simulink model "controller"  (R2025a)
settings: Solver=VariableStepAuto  StartTime=0.0  StopTime=20  RelTol=1e-3
values from neighbouring files (symbols this model uses):
  qd = [0 5.20948749525e-05 0.00020837949981 0.000468853874573 0.000833517999241 0.00130237187381 0.00187541549829 0.00255264887267 0.00333407199696 0.00421968487116 0.00520948749525 0.00630347986926 ... (2700 elements, 450x6)]    [dq.mat]
undefined symbols (not defined in the file or in its folder): D, ddqd, dqd, new_time, Q, rou
(part 1 of 2)
settings Model: Creator=CYX  LastModifiedBy=yxlewis
settings DebuggingCC: ParameterPrecisionLossMsg=none  UnderSpecifiedDimensionMsg=warning
settings RTWCC: GPUComputeCapability=3.5
settings SimscapeCC: SimscapeLogDecimation=1  SimscapeLogDataHistory=5000

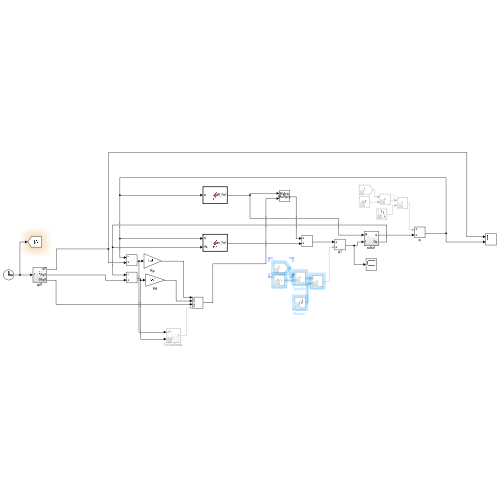
[thumbnail: Simulink's stored preview of the top-level diagram]
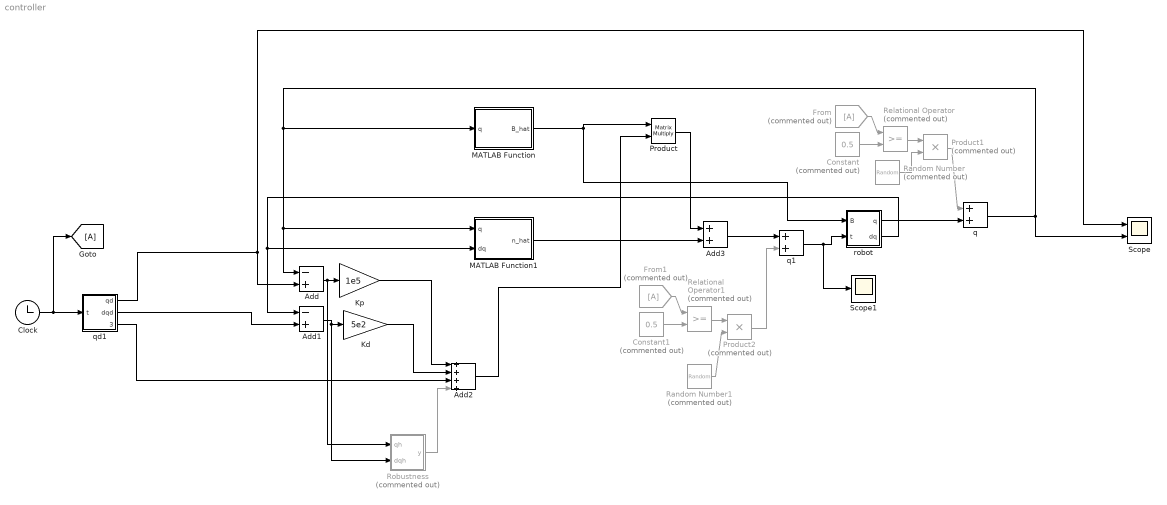
== system controller ==
  Add : Sum  Inputs=-+
  Add1 : Sum  Inputs=-+
  Add2 : Sum  Inputs=++++
  Add3 : Sum
  Clock : Clock
  Constant : Constant  Commented=on  Value=0.5
  Constant1 : Constant  Commented=on  Value=0.5
  From : From  Commented=on
  From1 : From  Commented=on
  Goto : Goto
  Kd : Gain  Gain=5e2
  Kp : Gain  Gain=1e5
  MATLAB Function : MATLAB Function  TreatAsAtomicUnit=on
  MATLAB Function1 : MATLAB Function  TreatAsAtomicUnit=on
  Product : Product  Multiplication=Matrix(*)
  Product1 : Product  Commented=on
  Product2 : Product  Commented=on
  Random Number : RandomNumber  Commented=on  Variance=1e-4  SampleTime=1e-2
  Random Number1 : RandomNumber  Commented=on  Variance=1e-4  SampleTime=1e-2
  Relational Operator : RelationalOperator  Commented=on  OutDataTypeStr=boolean  RndMeth=Simplest  InputSameDT=off
  Relational Operator1 : RelationalOperator  Commented=on  OutDataTypeStr=boolean  RndMeth=Simplest  InputSameDT=off
  Robustness : Subsystem  Commented=on
  Scope : Scope  NumInputPorts=2
      settings: ActiveDisplayYMinimum=-4.68170124056776  ActiveDisplayYMaximum=3.2186322366566769
  Scope1 : Scope
      settings: ActiveDisplayYMinimum=-244.17864380949288  ActiveDisplayYMaximum=369.16272311248588
  q : Sum
  q1 : Sum
  qd1 : Subsystem
  robot : Subsystem
  wires:
  qd1/3(ddqd) -> Add2/3
  Robustness/1(y) -> Add2/4
  Add2/1 -> Product/2
  Kp/1 -> Add2/1
  Add/1 -> Robustness/1(qh), Kp/1
  Product/1 -> Add3/1
  qd1/2(dqd) -> Add1/2
  MATLAB Function/1(B_hat) -> Product/1, robot/1(B)
  qd1/1(qd) -> Scope/1, Add/2
  Add1/1 -> Robustness/2(dqh), Kd/1
  Kd/1 -> Add2/2
  MATLAB Function1/1(n_hat) -> Add3/2
  Clock/1 -> qd1/1(t), Goto/1
  robot/2(dq) -> Add1/1, MATLAB Function1/2(dq)
  robot/1(q) -> q/2
  q/1 -> Scope/2, MATLAB Function/1(q), MATLAB Function1/1(q), Add/1
  Add3/1 -> q1/1
  q1/1 -> Scope1/1, robot/2(t)
  Constant/1 -> Relational Operator/2
  From/1 -> Relational Operator/1
  Relational Operator/1 -> Product1/1
  Random Number/1 -> Product1/2
  Product1/1 -> q/1
  Relational Operator1/1 -> Product2/1
  From1/1 -> Relational Operator1/1
  Constant1/1 -> Relational Operator1/2
  Random Number1/1 -> Product2/2
  Product2/1 -> q1/2

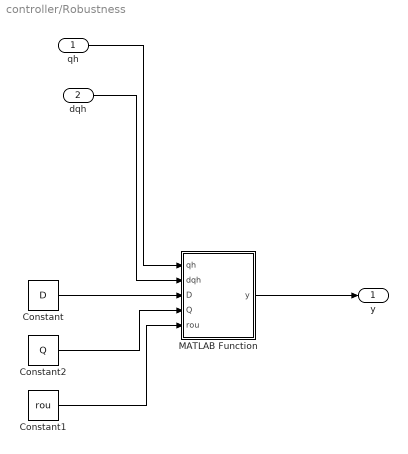
== system controller/Robustness ==
  qh : Inport
  dqh : Inport  Port=2
  Constant : Constant  Value=D
  Constant1 : Constant  Value=rou
  Constant2 : Constant  Value=Q
  MATLAB Function : MATLAB Function  TreatAsAtomicUnit=on
  y : Outport
  wires:
  Constant2/1 -> MATLAB Function/4(Q)
  dqh/1 -> MATLAB Function/2(dqh)
  qh/1 -> MATLAB Function/1(qh)
  MATLAB Function/1(y) -> y/1
  Constant/1 -> MATLAB Function/3(D)
  Constant1/1 -> MATLAB Function/5(rou)

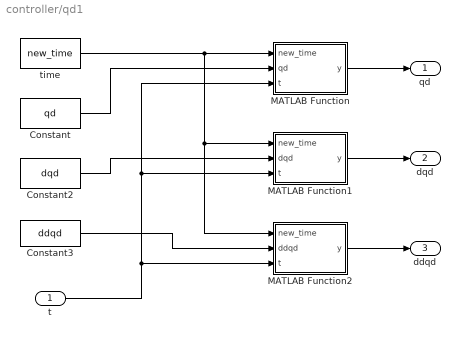
== system controller/qd1 ==
  t : Inport
  Constant : Constant  Value=qd
  Constant2 : Constant  Value=dqd
  Constant3 : Constant  Value=ddqd
  MATLAB Function : MATLAB Function  TreatAsAtomicUnit=on
  MATLAB Function1 : MATLAB Function  TreatAsAtomicUnit=on
  MATLAB Function2 : MATLAB Function  TreatAsAtomicUnit=on
  time : Constant  Value=new_time
  qd : Outport  PortDimensions=6*1
  dqd : Outport  Port=2  PortDimensions=6*1
  ddqd : Outport  Port=3  PortDimensions=6*1
  wires:
  time/1 -> MATLAB Function2/1(new_time), MATLAB Function1/1(new_time), MATLAB Function/1(new_time)
  Constant/1 -> MATLAB Function/2(qd)
  t/1 -> MATLAB Function2/3(t), MATLAB Function1/3(t), MATLAB Function/3(t)
  Constant2/1 -> MATLAB Function1/2(dqd)
  Constant3/1 -> MATLAB Function2/2(ddqd)
  MATLAB Function/1(y) -> qd/1
  MATLAB Function1/1(y) -> dqd/1
  MATLAB Function2/1(y) -> ddqd/1

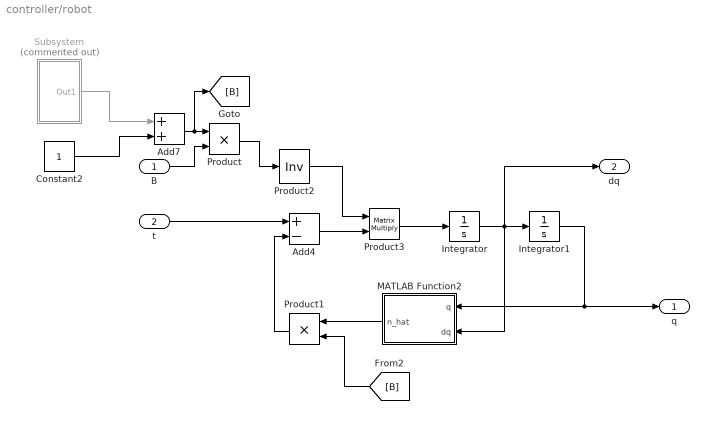
== system controller/robot ==
  B : Inport
  t : Inport  Port=2
  Add4 : Sum  Inputs=+-
  Add7 : Sum
  Constant2 : Constant
  Integrator : Integrator
  Integrator1 : Integrator
  MATLAB Function2 : MATLAB Function  TreatAsAtomicUnit=on
  Product : Product
  Product1 : Product
  Product2 : Product  Inputs=/  Multiplication=Matrix(*)
  Product3 : Product  Multiplication=Matrix(*)
  Subsystem : Subsystem  Commented=on
  q : Outport
  dq : Outport  Port=2
  wires:
  Integrator/1 -> dq/1, MATLAB Function2/2(dq), Integrator1/1
  t/1 -> Add4/1
  Product3/1 -> Integrator/1
  Integrator1/1 -> q/1, MATLAB Function2/1(q)
  Product2/1 -> Product3/1
  Add4/1 -> Product3/2
  MATLAB Function2/1(n_hat) -> Product1/1
  Product1/1 -> Add4/2
  Product/1 -> Product2/1
  Constant2/1 -> Add7/2
  Add7/1 -> [B], Product/1
  B/1 -> Product/2
  [B] -> Product1/2
  Subsystem/1(Out1) -> Add7/1

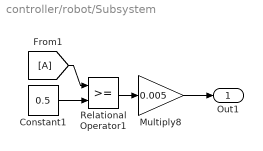
== system controller/robot/Subsystem ==
  Constant1 : Constant  Value=0.5
  From1 : From
  Multiply8 : Gain  Gain=0.005
  Relational Operator1 : RelationalOperator  OutDataTypeStr=boolean  RndMeth=Simplest  InputSameDT=off
  Out1 : Outport
  wires:
  From1/1 -> Relational Operator1/1
  Constant1/1 -> Relational Operator1/2
  Relational Operator1/1 -> Multiply8/1
  Multiply8/1 -> Out1/1

== matlab function controller/MATLAB Function1 ==
  data: q input size=6*1; n_hat output size=6*1; dq input size=6*1
function n_hat = fcn(q, dq)
th = q;
dth = dq;
th1 = th(1); th2 = th(2); th3 = th(3); th4 = th(4); th5 = th(5); th6 = th(6);
dth1 = dth(1); dth2 = dth(2); dth3 = dth(3); dth4 = dth(4); dth5 = dth(5); dth6 = dth(6);
% % ddth1 = ddth(1); ddth2 = ddth(2); ddth3 = ddth(3); ddth4 = ddth(4); ddth5 = ddth(5); ddth6 = ddth(6);

G = [0;
    (1866843*sin(th2 - th3 + th4 + th5))/2000000 - (795688119*sin(th2 - th3))/25000000 - (1866843*sin(th2 - th3 + th4 - th5))/2000000 - (40439763*sin(th2 - th3 + th4))/6250000 - (689642019*sin(th2))/12500000;
     (795688119*sin(th2 - th3))/25000000 - (1866843*sin(th2 - th3 + th4 + th5))/2000000 + (1866843*sin(th2 - th3 + th4 - th5))/2000000 + (40439763*sin(th2 - th3 + th4))/6250000;
     (1866843*sin(th2 - th3 + th4 + th5))/2000000 - (1866843*sin(th2 - th3 + th4 - th5))/2000000 - (40439763*sin(th2 - th3 + th4))/6250000;
     (1866843*sin(th2 - th3 + th4 + th5))/2000000 + (1866843*sin(th2 - th3 + th4 - th5))/2000000;
     0];

C = [(138917031*dth2^2*sin(th2))/250000000 - (5709*dth2^2*sin(th2 - th3 + th4 + th5))/2500000 - (5709*dth3^2*sin(th2 - th3 + th4 + th5))/2500000 - (5709*dth4^2*sin(th2 - th3 + th4 + th5))/2500000 - (173173*dth5^2*sin(th2 - th3 + th4 + th5))/5000000 + (2438609*dth2^2*sin(th2 - th3))/6250000 + (2438609*dth3^2*sin(th2 - th3))/6250000 + (378697*dth2^2*sin(th2 - th5))/10000000 - (378697*dth5^2*sin(th2 - th5))/10000000 + (173173*dth2^2*sin(th2 - th3 + th4 - th5))/5000000 + (2389*dth2^2*sin(th2 - th3 + th4 - 2*th5))/1250000 - (2389*dth2^2*sin(th2 - th3 + th4 + 2*th5))/1250000 + (173173*dth3^2*sin(th2 - th3 + th4 - th5))/5000000 + (2389*dth3^2*sin(th2 - th3 + th4 - 2*th5))/1250000 - (2389*dth3^2*sin(th2 - th3 + th4 + 2*th5))/1250000 + (173173*dth4^2*sin(th2 - th3 + th4 - th5))/5000000 + (2389*dth4^2*sin(th2 - th3 + th4 - 2*th5))/1250000 - (2389*dth4^2*sin(th2 - th3 + th4 + 2*th5))/1250000 + (5709*dth5^2*sin(th2 - th3 + th4 - th5))/2500000 + (3998631*dth2^2*sin(th2 - th3 + th4))/31250000 + (17127*dth2^2*sin(th2 - th3 + th5))/500000 - (17127*dth2^2*sin(th3 - th2 + th5))/500000 + (3998631*dth3^2*sin(th2 - th3 + th4))/31250000 + (17127*dth3^2*sin(th2 - th3 + th5))/500000 - (17127*dth3^2*sin(th3 - th2 + th5))/500000 + (3998631*dth4^2*sin(th2 - th3 + th4))/31250000 - (17127*dth5^2*sin(th2 - th3 + th5))/500000 + (17127*dth5^2*sin(th3 - th2 + th5))/500000 + (378697*dth2^2*sin(th2 + th5))/10000000 - (378697*dth5^2*sin(th2 + th5))/10000000 - (161408701*dth1*dth3*sin(th3))/125000000 - (371007*dth1*dth4*sin(th4))/1562500 - (184591*dth1*dth5*sin(th5))/2500000 + (8203377*dth1*dth2*sin(2*th2 - th3 + th4))/15625000 + (371007*dth1*dth2*sin(2*th2 - 2*th3 + th4))/781250 - (8203377*dth1*dth3*sin(2*th2 - th3 + th4))/31250000 - (371007*dth1*dth3*sin(2*th2 - 2*th3 + th4))/781250 + (8203377*dth1*dth4*sin(2*th2 - th3 + th4))/31250000 + (371007*dth1*dth4*sin(2*th2 - 2*th3 + th4))/1562500 + (5709*dth2*dth3*sin(th2 - th3 + th4 + th5))/1250000 - (5709*dth2*dth4*sin(th2 - th3 + th4 + th5))/1250000 - (184591*dth2*dth5*sin(th2 - th3 + th4 + th5))/5000000 + (5709*dth3*dth4*sin(th2 - th3 + th4 + th5))/1250000 + (dth2*dth6*sin(th2 - th3 + th4 + th5))/20000 + (184591*dth3*dth5*sin(th2 - th3 + th4 + th5))/5000000 - (dth3*dth6*sin(th2 - th3 + th4 + th5))/20000 - (184591*dth4*dth5*sin(th2 - th3 + th4 + th5))/5000000 + (dth4*dth6*sin(th2 - th3 + th4 + th5))/20000 + (dth5*dth6*sin(th2 - th3 + th4 + th5))/20000 - (2438609*dth2*dth3*sin(th2 - th3))/3125000 - (8203377*dth1*dth3*sin(th3 - th4))/31250000 + (8203377*dth1*dth4*sin(th3 - th4))/31250000 - (17127*dth1*dth4*sin(th4 - th5))/500000 + (17127*dth1*dth5*sin(th4 - th5))/500000 + (32351*dth1*dth2*sin(2*th2 - 2*th3 + 2*th4 - th5))/1000000 + (2389*dth1*dth2*sin(2*th2 - 2*th3 + 2*th4 - 2*th5))/1250000 + (2389*dth1*dth2*sin(2*th2 - 2*th3 + 2*th4 + 2*th5))/1250000 - (32351*dth1*dth3*sin(2*th2 - 2*th3 + 2*th4 - th5))/1000000 - (2389*dth1*dth3*sin(2*th2 - 2*th3 + 2*th4 - 2*th5))/1250000 - (2389*dth1*dth3*sin(2*th2 - 2*th3 + 2*th4 + 2*th5))/1250000 + (32351*dth1*dth4*sin(2*th2 - 2*th3 + 2*th4 - th5))/1000000 + (2389*dth1*dth4*sin(2*th2 - 2*th3 + 2*th4 - 2*th5))/1250000 + (2389*dth1*dth4*sin(2*th2 - 2*th3 + 2*th4 + 2*th5))/1250000 - (32351*dth1*dth5*sin(2*th2 - 2*th3 + 2*th4 - th5))/2000000 - (2389*dth1*dth5*sin(2*th2 - 2*th3 + 2*th4 - 2*th5))/1250000 + (2389*dth1*dth5*sin(2*th2 - 2*th3 + 2*th4 + 2*th5))/1250000 + (212507419*dth1*dth2*sin(2*th2))/125000000 - (2389*dth1*dth5*sin(2*th5))/625000 + (526847*dth1*dth2*sin(2*th2 - 2*th3 + 2*th4))/6250000 - (526847*dth1*dth3*sin(2*th2 - 2*th3 + 2*th4))/6250000 + (526847*dth1*dth4*sin(2*th2 - 2*th3 + 2*th4))/6250000 - (378697*dth1*dth2*sin(2*th2 - th3 + th4 + th5))/5000000 - (17127*dth1*dth2*sin(2*th2 - 2*th3 + th4 + th5))/250000 + (378697*dth1*dth3*sin(2*th2 - th3 + th4 + th5))/10000000 - (173173*dth2*dth3*sin(th2 - th3 + th4 - th5))/2500000 + (17127*dth1*dth3*sin(2*th2 - 2*th3 + th4 + th5))/250000 - (378697*dth1*dth4*sin(2*th2 - th3 + th4 + th5))/10000000 - (2389*dth2*dth3*sin(th2 - th3 + th4 - 2*th5))/625000 + (2389*dth2*dth3*sin(th2 - th3 + th4 + 2*th5))/625000 + (173173*dth2*dth4*sin(th2 - th3 + th4 - th5))/2500000 - (17127*dth1*dth4*sin(2*th2 - 2*th3 + th4 + th5))/500000 - (378697*dth1*dth5*sin(2*th2 - th3 + th4 + th5))/10000000 + (2389*dth2*dth4*sin(th2 - th3 + th4 - 2*th5))/625000 - (2389*dth2*dth4*sin(th2 - th3 + th4 + 2*th5))/625000 - (184591*dth2*dth5*sin(th2 - th3 + th4 - th5))/5000000 - (173173*dth3*dth4*sin(th2 - th3 + th4 - th5))/2500000 - (17127*dth1*dth5*sin(2*th2 - 2*th3 + th4 + th5))/500000 - (2389*dth2*dth5*sin(th2 - th3 + th4 - 2*th5))/625000 - (2389*dth2*dth5*sin(th2 - th3 + th4 + 2*th5))/625000 - (dth2*dth6*sin(th2 - th3 + th4 - th5))/20000 - (2389*dth3*dth4*sin(th2 - th3 + th4 - 2*th5))/625000 + (2389*dth3*dth4*sin(th2 - th3 + th4 + 2*th5))/625000 + (184591*dth3*dth5*sin(th2 - th3 + th4 - th5))/5000000 + (2389*dth3*dth5*sin(th2 - th3 + th4 - 2*th5))/625000 + (2389*dth3*dth5*sin(th2 - th3 + th4 + 2*th5))/625000 + (dth3*dth6*sin(th2 - th3 + th4 - th5))/20000 - (184591*dth4*dth5*sin(th2 - th3 + th4 - th5))/5000000 - (2389*dth4*dth5*sin(th2 - th3 + th4 - 2*th5))/625000 - (2389*dth4*dth5*sin(th2 - th3 + th4 + 2*th5))/625000 - (dth4*dth6*sin(th2 - th3 + th4 - th5))/20000 + (dth5*dth6*sin(th2 - th3 + th4 - th5))/20000 + (161408701*dth1*dth2*sin(2*th2 - th3))/62500000 + (509639*dth1*dth2*sin(2*th2 - 2*th3))/625000 - (161408701*dth1*dth3*sin(2*th2 - th3))/125000000 - (509639*dth1*dth3*sin(2*th2 - 2*th3))/625000 - (3998631*dth2*dth3*sin(th2 - th3 + th4))/15625000 - (17127*dth2*dth3*sin(th2 - th3 + th5))/250000 + (17127*dth2*dth3*sin(th3 - th2 + th5))/250000 + (3998631*dth2*dth4*sin(th2 - th3 + th4))/15625000 - (378697*dth1*dth3*sin(th3 - th4 + th5))/10000000 - (378697*dth1*dth3*sin(th4 - th3 + th5))/10000000 - (13431*dth2*dth5*sin(th2 - th3 + th4))/1250000 - (3998631*dth3*dth4*sin(th2 - th3 + th4))/15625000 + (378697*dth1*dth4*sin(th3 - th4 + th5))/10000000 + (378697*dth1*dth4*sin(th4 - th3 + th5))/10000000 + (13431*dth3*dth5*sin(th2 - th3 + th4))/1250000 - (378697*dth1*dth5*sin(th3 - th4 + th5))/10000000 + (378697*dth1*dth5*sin(th4 - th3 + th5))/10000000 - (13431*dth4*dth5*sin(th2 - th3 + th4))/1250000 + (17127*dth1*dth4*sin(th4 + th5))/500000 + (17127*dth1*dth5*sin(th4 + th5))/500000 + (378697*dth1*dth2*sin(2*th2 - th3 + th4 - th5))/5000000 + (17127*dth1*dth2*sin(2*th2 - 2*th3 + th4 - th5))/250000 - (378697*dth1*dth3*sin(2*th2 - th3 + th4 - th5))/10000000 - (32351*dth1*dth2*sin(2*th2 - 2*th3 + 2*th4 + th5))/1000000 - (17127*dth1*dth3*sin(2*th2 - 2*th3 + th4 - th5))/250000 + (378697*dth1*dth4*sin(2*th2 - th3 + th4 - th5))/10000000 + (32351*dth1*dth3*sin(2*th2 - 2*th3 + 2*th4 + th5))/1000000 + (17127*dth1*dth4*sin(2*th2 - 2*th3 + th4 - th5))/500000 - (378697*dth1*dth5*sin(2*th2 - th3 + th4 - th5))/10000000 - (32351*dth1*dth4*sin(2*th2 - 2*th3 + 2*th4 + th5))/1000000 - (17127*dth1*dth5*sin(2*th2 - 2*th3 + th4 - th5))/500000 - (32351*dth1*dth5*sin(2*th2 - 2*th3 + 2*th4 + th5))/2000000;
(161408701*dth3^2*sin(th3))/125000000 - (371007*dth4^2*sin(th4))/1562500 + (32351*dth5^2*sin(th5))/1000000 - (8203377*dth1^2*sin(2*th2 - th3 + th4))/31250000 - (371007*dth1^2*sin(2*th2 - 2*th3 + th4))/1562500 + (8203377*dth3^2*sin(th3 - th4))/31250000 + (8203377*dth4^2*sin(th3 - th4))/31250000 - (17127*dth4^2*sin(th4 - th5))/500000 - (17127*dth5^2*sin(th4 - th5))/500000 - (32351*dth1^2*sin(2*th2 - 2*th3 + 2*th4 - th5))/2000000 - (2389*dth1^2*sin(2*th2 - 2*th3 + 2*th4 - 2*th5))/2500000 - (2389*dth1^2*sin(2*th2 - 2*th3 + 2*th4 + 2*th5))/2500000 - (212507419*dth1^2*sin(2*th2))/250000000 - (526847*dth1^2*sin(2*th2 - 2*th3 + 2*th4))/12500000 + (378697*dth1^2*sin(2*th2 - th3 + th4 + th5))/10000000 + (17127*dth1^2*sin(2*th2 - 2*th3 + th4 + th5))/500000 - (161408701*dth1^2*sin(2*th2 - th3))/125000000 - (509639*dth1^2*sin(2*th2 - 2*th3))/1250000 + (378697*dth3^2*sin(th3 - th4 + th5))/10000000 + (378697*dth3^2*sin(th4 - th3 + th5))/10000000 + (378697*dth4^2*sin(th3 - th4 + th5))/10000000 + (378697*dth4^2*sin(th4 - th3 + th5))/10000000 + (378697*dth5^2*sin(th3 - th4 + th5))/10000000 + (378697*dth5^2*sin(th4 - th3 + th5))/10000000 + (17127*dth4^2*sin(th4 + th5))/500000 + (17127*dth5^2*sin(th4 + th5))/500000 - (378697*dth1^2*sin(2*th2 - th3 + th4 - th5))/10000000 - (17127*dth1^2*sin(2*th2 - 2*th3 + th4 - th5))/500000 + (32351*dth1^2*sin(2*th2 - 2*th3 + 2*th4 + th5))/2000000 - (161408701*dth2*dth3*sin(th3))/62500000 - (371007*dth2*dth4*sin(th4))/781250 + (371007*dth3*dth4*sin(th4))/781250 - (dth5*dth6*sin(th5))/10000 + (32351*dth1*dth5*sin(th2 - th3 + th4 + th5))/1000000 - (dth1*dth6*sin(th2 - th3 + th4 + th5))/20000 - (8203377*dth2*dth3*sin(th3 - th4))/15625000 - (378697*dth1*dth5*sin(th2 - th5))/5000000 + (8203377*dth2*dth4*sin(th3 - th4))/15625000 - (8203377*dth3*dth4*sin(th3 - th4))/15625000 - (17127*dth2*dth4*sin(th4 - th5))/250000 + (17127*dth2*dth5*sin(th4 - th5))/250000 + (17127*dth3*dth4*sin(th4 - th5))/250000 - (17127*dth3*dth5*sin(th4 - th5))/250000 + (17127*dth4*dth5*sin(th4 - th5))/250000 + (2389*dth2*dth5*sin(2*th5))/312500 - (2389*dth3*dth5*sin(2*th5))/312500 + (2389*dth4*dth5*sin(2*th5))/312500 - (32351*dth1*dth5*sin(th2 - th3 + th4 - th5))/1000000 - (2389*dth1*dth5*sin(th2 - th3 + th4 - 2*th5))/625000 - (2389*dth1*dth5*sin(th2 - th3 + th4 + 2*th5))/625000 + (dth1*dth6*sin(th2 - th3 + th4 - th5))/20000 + (13431*dth1*dth5*sin(th2 - th3 + th4))/1250000 + (17127*dth1*dth5*sin(th2 - th3 + th5))/250000 + (17127*dth1*dth5*sin(th3 - th2 + th5))/250000 - (378697*dth2*dth3*sin(th3 - th4 + th5))/5000000 - (378697*dth2*dth3*sin(th4 - th3 + th5))/5000000 + (378697*dth2*dth4*sin(th3 - th4 + th5))/5000000 + (378697*dth2*dth4*sin(th4 - th3 + th5))/5000000 - (378697*dth2*dth5*sin(th3 - th4 + th5))/5000000 + (378697*dth2*dth5*sin(th4 - th3 + th5))/5000000 - (378697*dth3*dth4*sin(th3 - th4 + th5))/5000000 - (378697*dth3*dth4*sin(th4 - th3 + th5))/5000000 + (378697*dth3*dth5*sin(th3 - th4 + th5))/5000000 - (378697*dth3*dth5*sin(th4 - th3 + th5))/5000000 - (378697*dth4*dth5*sin(th3 - th4 + th5))/5000000 + (378697*dth4*dth5*sin(th4 - th3 + th5))/5000000 + (378697*dth1*dth5*sin(th2 + th5))/5000000 + (17127*dth2*dth4*sin(th4 + th5))/250000 + (17127*dth2*dth5*sin(th4 + th5))/250000 - (17127*dth3*dth4*sin(th4 + th5))/250000 - (17127*dth3*dth5*sin(th4 + th5))/250000 + (17127*dth4*dth5*sin(th4 + th5))/250000;
(161408701*dth1^2*sin(th3))/250000000 + (161408701*dth2^2*sin(th3))/125000000 + (371007*dth4^2*sin(th4))/1562500 - (32351*dth5^2*sin(th5))/1000000 + (8203377*dth1^2*sin(2*th2 - th3 + th4))/62500000 + (371007*dth1^2*sin(2*th2 - 2*th3 + th4))/1562500 + (8203377*dth1^2*sin(th3 - th4))/62500000 + (8203377*dth2^2*sin(th3 - th4))/31250000 + (17127*dth4^2*sin(th4 - th5))/500000 + (17127*dth5^2*sin(th4 - th5))/500000 + (32351*dth1^2*sin(2*th2 - 2*th3 + 2*th4 - th5))/2000000 + (2389*dth1^2*sin(2*th2 - 2*th3 + 2*th4 - 2*th5))/2500000 + (2389*dth1^2*sin(2*th2 - 2*th3 + 2*th4 + 2*th5))/2500000 + (526847*dth1^2*sin(2*th2 - 2*th3 + 2*th4))/12500000 - (378697*dth1^2*sin(2*th2 - th3 + th4 + th5))/20000000 - (17127*dth1^2*sin(2*th2 - 2*th3 + th4 + th5))/500000 + (161408701*dth1^2*sin(2*th2 - th3))/250000000 + (509639*dth1^2*sin(2*th2 - 2*th3))/1250000 + (378697*dth1^2*sin(th3 - th4 + th5))/20000000 + (378697*dth1^2*sin(th4 - th3 + th5))/20000000 + (378697*dth2^2*sin(th3 - th4 + th5))/10000000 + (378697*dth2^2*sin(th4 - th3 + th5))/10000000 - (17127*dth4^2*sin(th4 + th5))/500000 - (17127*dth5^2*sin(th4 + th5))/500000 + (378697*dth1^2*sin(2*th2 - th3 + th4 - th5))/20000000 + (17127*dth1^2*sin(2*th2 - 2*th3 + th4 - th5))/500000 - (32351*dth1^2*sin(2*th2 - 2*th3 + 2*th4 + th5))/2000000 + (371007*dth2*dth4*sin(th4))/781250 - (371007*dth3*dth4*sin(th4))/781250 + (dth5*dth6*sin(th5))/10000 - (32351*dth1*dth5*sin(th2 - th3 + th4 + th5))/1000000 + (dth1*dth6*sin(th2 - th3 + th4 + th5))/20000 + (17127*dth2*dth4*sin(th4 - th5))/250000 - (17127*dth2*dth5*sin(th4 - th5))/250000 - (17127*dth3*dth4*sin(th4 - th5))/250000 + (17127*dth3*dth5*sin(th4 - th5))/250000 - (17127*dth4*dth5*sin(th4 - th5))/250000 - (2389*dth2*dth5*sin(2*th5))/312500 + (2389*dth3*dth5*sin(2*th5))/312500 - (2389*dth4*dth5*sin(2*th5))/312500 + (32351*dth1*dth5*sin(th2 - th3 + th4 - th5))/1000000 + (2389*dth1*dth5*sin(th2 - th3 + th4 - 2*th5))/625000 + (2389*dth1*dth5*sin(th2 - th3 + th4 + 2*th5))/625000 - (dth1*dth6*sin(th2 - th3 + th4 - th5))/20000 - (13431*dth1*dth5*sin(th2 - th3 + th4))/1250000 - (17127*dth1*dth5*sin(th2 - th3 + th5))/250000 - (17127*dth1*dth5*sin(th3 - th2 + th5))/250000 - (17127*dth2*dth4*sin(th4 + th5))/250000 - (17127*dth2*dth5*sin(th4 + th5))/250000 + (17127*dth3*dth4*sin(th4 + th5))/250000 + (17127*dth3*dth5*sin(th4 + th5))/250000 - (17127*dth4*dth5*sin(th4 + th5))/250000;
(371007*dth1^2*sin(th4))/3125000 + (371007*dth2^2*sin(th4))/1562500 + (371007*dth3^2*sin(th4))/1562500 + (32351*dth5^2*sin(th5))/1000000 - (8203377*dth1^2*sin(2*th2 - th3 + th4))/62500000 - (371007*dth1^2*sin(2*th2 - 2*th3 + th4))/3125000 - (8203377*dth1^2*sin(th3 - th4))/62500000 - (8203377*dth2^2*sin(th3 - th4))/31250000 + (17127*dth1^2*sin(th4 - th5))/1000000 + (17127*dth2^2*sin(th4 - th5))/500000 + (17127*dth3^2*sin(th4 - th5))/500000 - (32351*dth1^2*sin(2*th2 - 2*th3 + 2*th4 - th5))/2000000 - (2389*dth1^2*sin(2*th2 - 2*th3 + 2*th4 - 2*th5))/2500000 - (2389*dth1^2*sin(2*th2 - 2*th3 + 2*th4 + 2*th5))/2500000 - (526847*dth1^2*sin(2*th2 - 2*th3 + 2*th4))/12500000 + (378697*dth1^2*sin(2*th2 - th3 + th4 + th5))/20000000 + (17127*dth1^2*sin(2*th2 - 2*th3 + th4 + th5))/1000000 - (378697*dth1^2*sin(th3 - th4 + th5))/20000000 - (378697*dth1^2*sin(th4 - th3 + th5))/20000000 - (378697*dth2^2*sin(th3 - th4 + th5))/10000000 - (378697*dth2^2*sin(th4 - th3 + th5))/10000000 - (17127*dth1^2*sin(th4 + th5))/1000000 - (17127*dth2^2*sin(th4 + th5))/500000 - (17127*dth3^2*sin(th4 + th5))/500000 - (378697*dth1^2*sin(2*th2 - th3 + th4 - th5))/20000000 - (17127*dth1^2*sin(2*th2 - 2*th3 + th4 - th5))/1000000 + (32351*dth1^2*sin(2*th2 - 2*th3 + 2*th4 + th5))/2000000 - (371007*dth2*dth3*sin(th4))/781250 - (dth5*dth6*sin(th5))/10000 + (32351*dth1*dth5*sin(th2 - th3 + th4 + th5))/1000000 - (dth1*dth6*sin(th2 - th3 + th4 + th5))/20000 - (17127*dth2*dth3*sin(th4 - th5))/250000 + (2389*dth2*dth5*sin(2*th5))/312500 - (2389*dth3*dth5*sin(2*th5))/312500 + (2389*dth4*dth5*sin(2*th5))/312500 - (32351*dth1*dth5*sin(th2 - th3 + th4 - th5))/1000000 - (2389*dth1*dth5*sin(th2 - th3 + th4 - 2*th5))/625000 - (2389*dth1*dth5*sin(th2 - th3 + th4 + 2*th5))/625000 + (dth1*dth6*sin(th2 - th3 + th4 - th5))/20000 + (13431*dth1*dth5*sin(th2 - th3 + th4))/1250000 + (17127*dth2*dth3*sin(th4 + th5))/250000;
(184591*dth1^2*sin(th5))/5000000 - (17127*dth1^2*sin(th4 - th5))/1000000 - (17127*dth2^2*sin(th4 - th5))/500000 - (17127*dth3^2*sin(th4 - th5))/500000 + (32351*dth1^2*sin(2*th2 - 2*th3 + 2*th4 - th5))/4000000 + (2389*dth1^2*sin(2*th2 - 2*th3 + 2*th4 - 2*th5))/2500000 - (2389*dth1^2*sin(2*th2 - 2*th3 + 2*th4 + 2*th5))/2500000 + (2389*dth1^2*sin(2*th5))/1250000 - (2389*dth2^2*sin(2*th5))/625000 - (2389*dth3^2*sin(2*th5))/625000 - (2389*dth4^2*sin(2*th5))/625000 + (378697*dth1^2*sin(2*th2 - th3 + th4 + th5))/20000000 + (17127*dth1^2*sin(2*th2 - 2*th3 + th4 + th5))/1000000 + (378697*dth1^2*sin(th3 - th4 + th5))/20000000 - (378697*dth1^2*sin(th4 - th3 + th5))/20000000 + (378697*dth2^2*sin(th3 - th4 + th5))/10000000 - (378697*dth2^2*sin(th4 - th3 + th5))/10000000 - (17127*dth1^2*sin(th4 + th5))/1000000 - (17127*dth2^2*sin(th4 + th5))/500000 - (17127*dth3^2*sin(th4 + th5))/500000 + (378697*dth1^2*sin(2*th2 - th3 + th4 - th5))/20000000 + (17127*dth1^2*sin(2*th2 - 2*th3 + th4 - th5))/1000000 + (32351*dth1^2*sin(2*th2 - 2*th3 + 2*th4 + th5))/4000000 + (dth2*dth6*sin(th5))/10000 - (dth3*dth6*sin(th5))/10000 + (dth4*dth6*sin(th5))/10000 - (32351*dth1*dth2*sin(th2 - th3 + th4 + th5))/1000000 + (32351*dth1*dth3*sin(th2 - th3 + th4 + th5))/1000000 - (32351*dth1*dth4*sin(th2 - th3 + th4 + th5))/1000000 - (dth1*dth6*sin(th2 - th3 + th4 + th5))/20000 + (378697*dth1*dth2*sin(th2 - th5))/5000000 + (17127*dth2*dth3*sin(th4 - th5))/250000 + (2389*dth2*dth3*sin(2*th5))/312500 - (2389*dth2*dth4*sin(2*th5))/312500 + (2389*dth3*dth4*sin(2*th5))/312500 + (32351*dth1*dth2*sin(th2 - th3 + th4 - th5))/1000000 + (2389*dth1*dth2*sin(th2 - th3 + th4 - 2*th5))/625000 + (2389*dth1*dth2*sin(th2 - th3 + th4 + 2*th5))/625000 - (32351*dth1*dth3*sin(th2 - th3 + th4 - th5))/1000000 - (2389*dth1*dth3*sin(th2 - th3 + th4 - 2*th5))/625000 - (2389*dth1*dth3*sin(th2 - th3 + th4 + 2*th5))/625000 + (32351*dth1*dth4*sin(th2 - th3 + th4 - th5))/1000000 + (2389*dth1*dth4*sin(th2 - th3 + th4 - 2*th5))/625000 + (2389*dth1*dth4*sin(th2 - th3 + th4 + 2*th5))/625000 - (dth1*dth6*sin(th2 - th3 + th4 - th5))/20000 - (13431*dth1*dth2*sin(th2 - th3 + th4))/1250000 - (17127*dth1*dth2*sin(th2 - th3 + th5))/250000 - (17127*dth1*dth2*sin(th3 - th2 + th5))/250000 + (13431*dth1*dth3*sin(th2 - th3 + th4))/1250000 + (17127*dth1*dth3*sin(th2 - th3 + th5))/250000 + (17127*dth1*dth3*sin(th3 - th2 + th5))/250000 - (13431*dth1*dth4*sin(th2 - th3 + th4))/1250000 - (378697*dth1*dth2*sin(th2 + th5))/5000000 + (17127*dth2*dth3*sin(th4 + th5))/250000;
0];

n_hat = zeros(6,1);

n_hat = C+G;

== matlab function controller/MATLAB Function ==
  data: q input; B_hat output
function B_hat = fcn(q)
th = q;
th1 = th(1); th2 = th(2); th3 = th(3); th4 = th(4); th5 = th(5); th6 = th(6);

M = zeros(6,6);
M(:,1) = [(8203377*cos(th3 - th4))/31250000 + (17127*cos(th4 - th5))/500000 - (32351*cos(2*th2 - 2*th3 + 2*th4 - th5))/2000000 - (2389*cos(2*th2 - 2*th3 + 2*th4 - 2*th5))/2500000 - (2389*cos(2*th2 - 2*th3 + 2*th4 + 2*th5))/2500000 - (212507419*cos(2*th2))/250000000 + (2389*cos(2*th5))/1250000 - (526847*cos(2*th2 - 2*th3 + 2*th4))/12500000 + (378697*cos(2*th2 - th3 + th4 + th5))/10000000 + (17127*cos(2*th2 - 2*th3 + th4 + th5))/500000 - (161408701*cos(2*th2 - th3))/125000000 - (509639*cos(2*th2 - 2*th3))/1250000 + (378697*cos(th3 - th4 + th5))/10000000 - (378697*cos(th4 - th3 + th5))/10000000 - (17127*cos(th4 + th5))/500000 - (378697*cos(2*th2 - th3 + th4 - th5))/10000000 - (17127*cos(2*th2 - 2*th3 + th4 - th5))/500000 + (32351*cos(2*th2 - 2*th3 + 2*th4 + th5))/2000000 + (161408701*cos(th3))/125000000 + (371007*cos(th4))/1562500 + (184591*cos(th5))/2500000 - (8203377*cos(2*th2 - th3 + th4))/31250000 - (371007*cos(2*th2 - 2*th3 + th4))/1562500 + 7069546249637521/4503599627370496;
    (795688119*sin(th2 - th3))/25000000 - (378697*cos(th2 - th5))/10000000 - (40117736336437*cos(th3 - th2 - th4 + th5 + 6907208336974987/4503599627370496))/42949672960000 - (1866843*sin(th2 - th3 + th4 + th5))/2000000 - (3392996465943579*cos(th2 - th3 + th4 - 6985187348444747/4503599627370496))/524288000000000 - (2389*cos(th2 - th3 + th4 - 2*th5))/1250000 + (2389*cos(th2 - th3 + th4 + 2*th5))/1250000 + (1866843*sin(th2 - th3 + th4 - th5))/2000000 - (17127*cos(th2 - th3 + th5))/500000 - (17127*cos(th3 - th2 + th5))/500000 + (40439763*sin(th2 - th3 + th4))/6250000 - (1807946865178317*cos(th2 - 878610060698491/562949953421312))/32768000000000 - (378697*cos(th2 + th5))/10000000 - (6675217259932483*cos(th3 - th2 + 877378793755287/562949953421312))/209715200000000 + (689642019*sin(th2))/12500000 + (5011283516754143*cos(th2 - th3 + th4 + th5 - 7063219793270517/4503599627370496))/5368709120000000;
    (1866843*sin(th2 - th3 + th4 + th5))/2000000 + (40117736336437*cos(th3 - th2 - th4 + th5 + 6907208336974987/4503599627370496))/42949672960000 - (795688119*sin(th2 - th3))/25000000 + (3392996465943579*cos(th2 - th3 + th4 - 6985187348444747/4503599627370496))/524288000000000 + (2389*cos(th2 - th3 + th4 - 2*th5))/1250000 - (2389*cos(th2 - th3 + th4 + 2*th5))/1250000 - (1866843*sin(th2 - th3 + th4 - th5))/2000000 + (17127*cos(th2 - th3 + th5))/500000 + (17127*cos(th3 - th2 + th5))/500000 - (40439763*sin(th2 - th3 + th4))/6250000 + (6675217259932483*cos(th3 - th2 + 877378793755287/562949953421312))/209715200000000 - (5011283516754143*cos(th2 - th3 + th4 + th5 - 7063219793270517/4503599627370496))/5368709120000000;
    (2389*cos(th2 - th3 + th4 + 2*th5))/1250000 - (40117736336437*cos(th3 - th2 - th4 + th5 + 6907208336974987/4503599627370496))/42949672960000 - (3392996465943579*cos(th2 - th3 + th4 - 6985187348444747/4503599627370496))/524288000000000 - (2389*cos(th2 - th3 + th4 - 2*th5))/1250000 - (1866843*sin(th2 - th3 + th4 + th5))/2000000 + (1866843*sin(th2 - th3 + th4 - th5))/2000000 + (40439763*sin(th2 - th3 + th4))/6250000 + (5011283516754143*cos(th2 - th3 + th4 + th5 - 7063219793270517/4503599627370496))/5368709120000000;
    (5011283516754143*cos(th3 - th2 - th4 + th5 + 7063219793270517/4503599627370496))/5368709120000000 - (378697*cos(th2 - th5))/10000000 - (1866843*sin(th2 - th3 + th4 + th5))/2000000 - (1866843*sin(th2 - th3 + th4 - th5))/2000000 + (13431*cos(th2 - th3 + th4))/1250000 + (17127*cos(th2 - th3 + th5))/500000 - (17127*cos(th3 - th2 + th5))/500000 + (378697*cos(th2 + th5))/10000000 + (40117736336437*cos(th2 - th3 + th4 + th5 - 6907208336974987/4503599627370496))/42949672960000;
    cos(th2 - th3 + th4 - th5)/20000 - cos(th2 - th3 + th4 + th5)/20000];
M(:,2) = [(2389*cos(th2 - th3 + th4 + 2*th5))/1250000 - (378697*cos(th2 - th5))/10000000 - (173173*cos(th2 - th3 + th4 - th5))/5000000 - (2389*cos(th2 - th3 + th4 - 2*th5))/1250000 - (2438609*cos(th2 - th3))/6250000 - (3998631*cos(th2 - th3 + th4))/31250000 - (17127*cos(th2 - th3 + th5))/500000 - (17127*cos(th3 - th2 + th5))/500000 - (378697*cos(th2 + th5))/10000000 - (138917031*cos(th2))/250000000 + (5709*cos(th2 - th3 + th4 + th5))/2500000;
    (795688119*sin(th2 - th3))/25000000 - (1866843*sin(th2 - th3 + th4 + th5))/2000000 + (1866843*sin(th2 - th3 + th4 - th5))/2000000 + (40439763*sin(th2 - th3 + th4))/6250000 + (161408701*cos(th3))/62500000 + (371007*cos(th4))/781250 + (8203377*cos(th3)*cos(th4))/15625000 + (795688119*cos(th2)*sin(th3))/25000000 - (795688119*cos(th3)*sin(th2))/25000000 + (8203377*sin(th3)*sin(th4))/15625000 + (17127*sin(th4)*sin(th5))/125000 - (2389*cos(th5)^2)/312500 + (378697*cos(th3)*sin(th4)*sin(th5))/2500000 - (378697*cos(th4)*sin(th3)*sin(th5))/2500000 - (40439763*sin(th2)*sin(th3)*sin(th4))/6250000 - (40439763*cos(th2)*cos(th3)*sin(th4))/6250000 + (40439763*cos(th2)*cos(th4)*sin(th3))/6250000 - (40439763*cos(th3)*cos(th4)*sin(th2))/6250000 + (1866843*cos(th2)*cos(th3)*cos(th4)*sin(th5))/1000000 + (1866843*cos(th2)*sin(th3)*sin(th4)*sin(th5))/1000000 - (1866843*cos(th3)*sin(th2)*sin(th4)*sin(th5))/1000000 + (1866843*cos(th4)*sin(th2)*sin(th3)*sin(th5))/1000000 + 1483004097808091/562949953421312;
    (1866843*sin(th2 - th3 + th4 + th5))/2000000 - (795688119*sin(th2 - th3))/25000000 - (1866843*sin(th2 - th3 + th4 - th5))/2000000 - (40439763*sin(th2 - th3 + th4))/6250000 - (161408701*cos(th3))/125000000 - (371007*cos(th4))/781250 - (8203377*cos(th3)*cos(th4))/31250000 - (795688119*cos(th2)*sin(th3))/25000000 + (795688119*cos(th3)*sin(th2))/25000000 - (8203377*sin(th3)*sin(th4))/31250000 - (17127*sin(th4)*sin(th5))/125000 + (2389*cos(th5)^2)/312500 - (378697*cos(th3)*sin(th4)*sin(th5))/5000000 + (378697*cos(th4)*sin(th3)*sin(th5))/5000000 + (40439763*sin(th2)*sin(th3)*sin(th4))/6250000 + (40439763*cos(th2)*cos(th3)*sin(th4))/6250000 - (40439763*cos(th2)*cos(th4)*sin(th3))/6250000 + (40439763*cos(th3)*cos(th4)*sin(th2))/6250000 - (1866843*cos(th2)*cos(th3)*cos(th4)*sin(th5))/1000000 - (1866843*cos(th2)*sin(th3)*sin(th4)*sin(th5))/1000000 + (1866843*cos(th3)*sin(th2)*sin(th4)*sin(th5))/1000000 - (1866843*cos(th4)*sin(th2)*sin(th3)*sin(th5))/1000000 - 4153602922761353/4503599627370496;
    (1866843*sin(th2 - th3 + th4 - th5))/2000000 - (1866843*sin(th2 - th3 + th4 + th5))/2000000 + (40439763*sin(th2 - th3 + th4))/6250000 + (371007*cos(th4))/1562500 + (8203377*cos(th3)*cos(th4))/31250000 + (8203377*sin(th3)*sin(th4))/31250000 + (17127*sin(th4)*sin(th5))/250000 - (2389*cos(th5)^2)/312500 + (378697*cos(th3)*sin(th4)*sin(th5))/5000000 - (378697*cos(th4)*sin(th3)*sin(th5))/5000000 - (40439763*sin(th2)*sin(th3)*sin(th4))/6250000 - (40439763*cos(th2)*cos(th3)*sin(th4))/6250000 + (40439763*cos(th2)*cos(th4)*sin(th3))/6250000 - (40439763*cos(th3)*cos(th4)*sin(th2))/6250000 + (1866843*cos(th2)*cos(th3)*cos(th4)*sin(th5))/1000000 + (1866843*cos(th2)*sin(th3)*sin(th4)*sin(th5))/1000000 - (1866843*cos(th3)*sin(th2)*sin(th4)*sin(th5))/1000000 + (1866843*cos(th4)*sin(th2)*sin(th3)*sin(th5))/1000000 + 3669991262679561/36028797018963968;
    - (1866843*sin(th2 - th3 + th4 + th5))/2000000 - (1866843*sin(th2 - th3 + th4 - th5))/2000000 - (1903*cos(th5)*(199*cos(th3 - th4) - 4905*sin(th2 - th3 + th4) + 180*cos(th4) + 85))/5000000;
    cos(th5)/10000];
M(:,3) = [(2438609*cos(th2 - th3))/6250000 + (173173*cos(th2 - th3 + th4 - th5))/5000000 + (2389*cos(th2 - th3 + th4 - 2*th5))/1250000 - (2389*cos(th2 - th3 + th4 + 2*th5))/1250000 + (3998631*cos(th2 - th3 + th4))/31250000 + (17127*cos(th2 - th3 + th5))/500000 + (17127*cos(th3 - th2 + th5))/500000 - (5709*cos(th2 - th3 + th4 + th5))/2500000;
    (795688119*sin(th2 - th3))/25000000 - (1866843*sin(th2 - th3 + th4 + th5))/2000000 + (1866843*sin(th2 - th3 + th4 - th5))/2000000 + (40439763*sin(th2 - th3 + th4))/6250000 - (161408701*cos(th3))/125000000 - (371007*cos(th4))/781250 - (8203377*cos(th3)*cos(th4))/31250000 + (795688119*cos(th2)*sin(th3))/25000000 - (795688119*cos(th3)*sin(th2))/25000000 - (8203377*sin(th3)*sin(th4))/31250000 - (17127*sin(th4)*sin(th5))/125000 + (2389*cos(th5)^2)/312500 - (378697*cos(th3)*sin(th4)*sin(th5))/5000000 + (378697*cos(th4)*sin(th3)*sin(th5))/5000000 - (40439763*sin(th2)*sin(th3)*sin(th4))/6250000 - (40439763*cos(th2)*cos(th3)*sin(th4))/6250000 + (40439763*cos(th2)*cos(th4)*sin(th3))/6250000 - (40439763*cos(th3)*cos(th4)*sin(th2))/6250000 + (1866843*cos(th2)*cos(th3)*cos(th4)*sin(th5))/1000000 + (1866843*cos(th2)*sin(th3)*sin(th4)*sin(th5))/1000000 - (1866843*cos(th3)*sin(th2)*sin(th4)*sin(th5))/1000000 + (1866843*cos(th4)*sin(th2)*sin(th3)*sin(th5))/1000000 - 4153602922761353/4503599627370496;
    (17127*cos(th4 - th5))/250000 - (2389*cos(2*th5))/625000 - (17127*cos(th4 + th5))/250000 + (371007*cos(th4))/781250 + 1034097090886423/1125899906842624;
    (2389*cos(2*th5))/625000 - (17127*cos(th4 - th5))/500000 + (17127*cos(th4 + th5))/500000 - (371007*cos(th4))/1562500 - 7064549577908547/72057594037927936;
    (1903*cos(th5)*(981*sin(th2 - th3 + th4) + 36*cos(th4) + 17))/1000000 - (1866843*sin(th2 - th3 + th4 - th5))/2000000 - (1866843*sin(th2 - th3 + th4 + th5))/2000000;
    -cos(th5)/10000];
M(:,4) = [(2389*cos(th2 - th3 + th4 + 2*th5))/1250000 - (2389*cos(th2 - th3 + th4 - 2*th5))/1250000 - (173173*cos(th2 - th3 + th4 - th5))/5000000 - (3998631*cos(th2 - th3 + th4))/31250000 + (5709*cos(th2 - th3 + th4 + th5))/2500000;
    (795688119*sin(th2 - th3))/25000000 - (1866843*sin(th2 - th3 + th4 + th5))/2000000 + (1866843*sin(th2 - th3 + th4 - th5))/2000000 + (40439763*sin(th2 - th3 + th4))/6250000 + (371007*cos(th4))/1562500 + (8203377*cos(th3)*cos(th4))/31250000 + (795688119*cos(th2)*sin(th3))/25000000 - (795688119*cos(th3)*sin(th2))/25000000 + (8203377*sin(th3)*sin(th4))/31250000 + (17127*sin(th4)*sin(th5))/250000 - (2389*cos(th5)^2)/312500 + (378697*cos(th3)*sin(th4)*sin(th5))/5000000 - (378697*cos(th4)*sin(th3)*sin(th5))/5000000 - (40439763*sin(th2)*sin(th3)*sin(th4))/6250000 - (40439763*cos(th2)*cos(th3)*sin(th4))/6250000 + (40439763*cos(th2)*cos(th4)*sin(th3))/6250000 - (40439763*cos(th3)*cos(th4)*sin(th2))/6250000 + (1866843*cos(th2)*cos(th3)*cos(th4)*sin(th5))/1000000 + (1866843*cos(th2)*sin(th3)*sin(th4)*sin(th5))/1000000 - (1866843*cos(th3)*sin(th2)*sin(th4)*sin(th5))/1000000 + (1866843*cos(th4)*sin(th2)*sin(th3)*sin(th5))/1000000 + 3669991262679561/36028797018963968;
    (2389*cos(2*th5))/625000 - (17127*cos(th4 - th5))/500000 + (17127*cos(th4 + th5))/500000 - (371007*cos(th4))/1562500 - 7064549577908547/72057594037927936;
    7064549577908547/72057594037927936 - (2389*cos(2*th5))/625000;
    (1903*cos(th5)*(981*sin(th2 - th3 + th4) - 17))/1000000 - (1866843*sin(th2 - th3 + th4 - th5))/2000000 - (1866843*sin(th2 - th3 + th4 + th5))/2000000;
    cos(th5)/10000];
M(:,5) = [(5709*cos(th2 - th3 + th4 - th5))/2500000 - (378697*cos(th2 - th5))/10000000 + (13431*cos(th2 - th3 + th4))/1250000 + (17127*cos(th2 - th3 + th5))/500000 - (17127*cos(th3 - th2 + th5))/500000 + (378697*cos(th2 + th5))/10000000 + (173173*cos(th2 - th3 + th4 + th5))/5000000;
    (795688119*sin(th2 - th3))/25000000 - (1866843*sin(th2 - th3 + th4 + th5))/2000000 + (1866843*sin(th2 - th3 + th4 - th5))/2000000 + (40439763*sin(th2 - th3 + th4))/6250000 - (32351*cos(th5))/1000000 - (17127*cos(th4)*cos(th5))/250000 + (795688119*cos(th2)*sin(th3))/25000000 - (795688119*cos(th3)*sin(th2))/25000000 - (378697*cos(th5)*sin(th3)*sin(th4))/5000000 - (40439763*sin(th2)*sin(th3)*sin(th4))/6250000 - (378697*cos(th3)*cos(th4)*cos(th5))/5000000 - (40439763*cos(th2)*cos(th3)*sin(th4))/6250000 + (40439763*cos(th2)*cos(th4)*sin(th3))/6250000 - (40439763*cos(th3)*cos(th4)*sin(th2))/6250000 + (1866843*cos(th2)*cos(th3)*cos(th4)*sin(th5))/1000000 + (1866843*cos(th2)*sin(th3)*sin(th4)*sin(th5))/1000000 - (1866843*cos(th3)*sin(th2)*sin(th4)*sin(th5))/1000000 + (1866843*cos(th4)*sin(th2)*sin(th3)*sin(th5))/1000000;
    (17127*cos(th4 - th5))/500000 + (17127*cos(th4 + th5))/500000 + (32351*cos(th5))/1000000;
    -(32351*cos(th5))/1000000;
    6193955491349825/576460752303423488;
    0];
M(:,6) = [cos(th2 - th3 + th4 - th5)/20000 - cos(th2 - th3 + th4 + th5)/20000;
    cos(th5)/10000;
    -cos(th5)/10000;
    cos(th5)/10000;
    0;
    1/10000];

B_hat = M;
